simulink model "Problem4"  (R2020a)
settings: Solver=VariableStepAuto  StartTime=0.0  StopTime=10.0  RelTol=1e-3
settings Model: Creator=tanu  LastModifiedBy=tanu

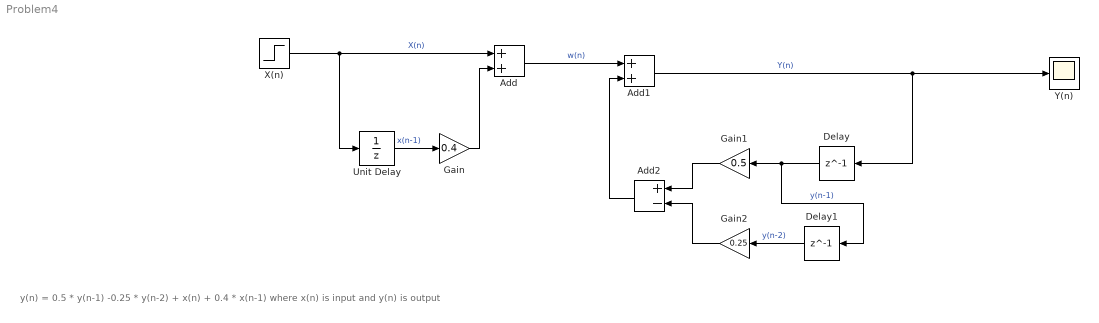
== system Problem4 ==
  note: y(n) = 0.5 * y(n-1) -0.25 * y(n-2) + x(n) + 0.4 * x(n-1)
      |
      | where x(n) is input and y(n) is output
  Add : Sum
  Add1 : Sum
  Add2 : Sum  Inputs=+-
  Delay : Delay  DelayLength=1
  Delay1 : Delay  DelayLength=1
  Gain : Gain  Gain=0.4
  Gain1 : Gain  Gain=0.5
  Gain2 : Gain  Gain=0.25
  Unit Delay : UnitDelay  SampleTime=-1  HasFrameUpgradeWarning=on
  X(n) : Step  SampleTime=0
  Y(n) : Scope
  wires:
  X(n)/1 -> Add/1, Unit Delay/1  "X(n)"
  Unit Delay/1 -> Gain/1  "x(n-1)"
  Gain/1 -> Add/2
  Add/1 -> Add1/1  "w(n)"
  Add1/1 -> Delay/1, Y(n)/1  "Y(n)"
  Delay/1 -> Delay1/1, Gain1/1  "y(n-1)"
  Delay1/1 -> Gain2/1  "y(n-2)"
  Gain1/1 -> Add2/1
  Gain2/1 -> Add2/2
  Add2/1 -> Add1/2
